simulink model "MBD_Math_Operations_1"  (R2021b)
settings: Solver=FixedStepDiscrete  StartTime=0.0  StopTime=10.0  FixedStep=0.0001  RelTol=1e-3
settings Model: Creator=waleed.elshemy  LastModifiedBy=waleed.elshemy
settings OptimizationCC: DefaultParameterBehavior=Inlined  UseDivisionForNetSlopeComputation=on  GainParamInheritBuiltInType=on  UseFloatMulNetSlope=on  InlineInvariantSignals=on  PassReuseOutputArgsAs=Individual arguments  ZeroExternalMemoryAtStartup=off  ZeroInternalMemoryAtStartup=off  NoFixptDivByZeroProtection=on  EfficientFloat2IntCast=on  LifeSpan=1  OptimizeBlockOrder=speed  DifferentSizesBufferReuse=on  EfficientTunableParamExpr=on
settings DebuggingCC: ParameterTunabilityLossMsg=error
settings HardwareCC: ProdLongLongMode=on
settings SFSimCC: MATLABDynamicMemAlloc=off
settings RTWCC: Description=Embedded Coder  SystemTargetFile=ert.tlc  TemplateMakefile=ert_default_tmf
settings CodeAppCC: ForceParamTrailComments=on  IgnoreCustomStorageClasses=off  OperatorAnnotations=on  SimulinkDataObjDesc=on  SFDataObjDesc=on  CustomSymbolStrGlobalVar=rt$N$M  CustomSymbolStrType=$N$M  CustomSymbolStrFcn=$N$M$F  CustomSymbolStrMacro=$N$M  InsertBlockDesc=on
settings ERTTargetCC: TargetLangStandard=C99 (ISO)  GenerateSampleERTMain=on  IncludeMdlTerminateFcn=off  CombineSignalStateStructs=on  SuppressErrorStatus=on  SupportAbsoluteTime=off  SupportComplex=off  InlinedParameterPlacement=NonHierarchical  ERTCustomFileTemplate=example_file_process.tlc  ERTFilePackagingFormat=CompactWithDataFile

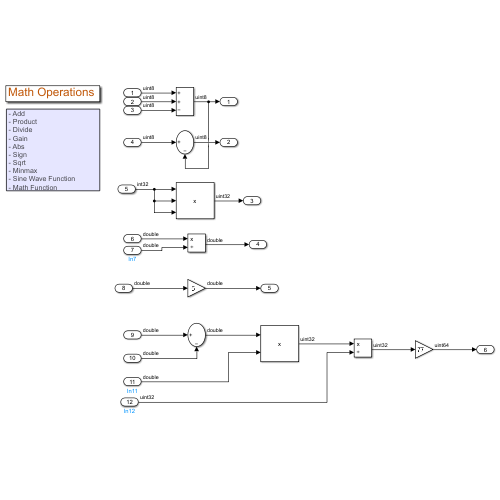
[thumbnail: Simulink's stored preview of the top-level diagram]
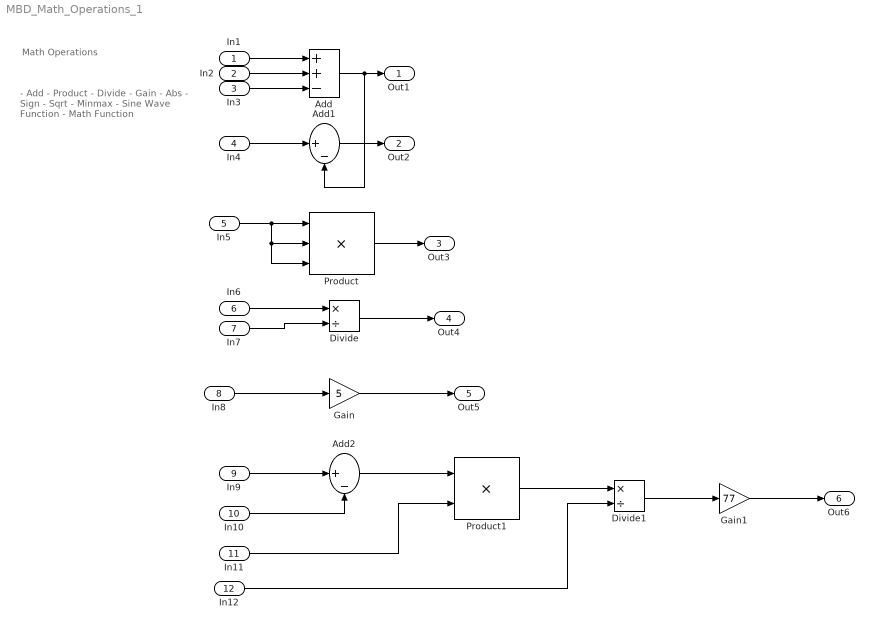
== system MBD_Math_Operations_1 ==
  note: - Add
      | - Product
      | - Divide
      | - Gain
      | - Abs
      | - Sign
      | - Sqrt
      | - Minmax
      | - Sine Wave Function
      | - Math Function
  note: Math Operations
  In1 : Inport
  In2 : Inport  Port=2
  In3 : Inport  Port=3
  In4 : Inport  Port=4  OutDataTypeStr=uint8
  In5 : Inport  Port=5  OutDataTypeStr=int32
  In6 : Inport  Port=6
  In7 : Inport  Port=7
  In8 : Inport  Port=8
  In9 : Inport  Port=9
  In10 : Inport  Port=10
  In11 : Inport  Port=11
  In12 : Inport  Port=12
  Add : Sum  Inputs=++-
  Add1 : Sum  Inputs=|+-
  Add2 : Sum  Inputs=|+-
  Divide : Product  Inputs=*/
  Divide1 : Product  Inputs=*/
  Gain : Gain  Gain=5
  Gain1 : Gain  Gain=77
  Product : Product  Inputs=3  OutDataTypeStr=uint32
  Product1 : Product  OutDataTypeStr=uint32
  Out1 : Outport
  Out2 : Outport  Port=2
  Out3 : Outport  Port=3
  Out4 : Outport  Port=4
  Out5 : Outport  Port=5
  Out6 : Outport  Port=6
  wires:
  In1/1 -> Add/1
  In2/1 -> Add/2
  In3/1 -> Add/3
  Add/1 -> Add1/2, Out1/1
  In4/1 -> Add1/1
  Add1/1 -> Out2/1
  In5/1 -> Product/2, Product/3, Product/1
  Product/1 -> Out3/1
  In6/1 -> Divide/1
  In7/1 -> Divide/2
  Divide/1 -> Out4/1
  In8/1 -> Gain/1
  Gain/1 -> Out5/1
  In9/1 -> Add2/1
  In10/1 -> Add2/2
  Add2/1 -> Product1/1
  In11/1 -> Product1/2
  Product1/1 -> Divide1/1
  In12/1 -> Divide1/2
  Divide1/1 -> Gain1/1
  Gain1/1 -> Out6/1
